simulink model "aimant_permanent_b"  (R2019a)
settings: Solver=VariableStepAuto  StartTime=0.0  StopTime=10.0  RelTol=1e-3
values from neighbouring files (symbols this model uses):
  Tl = 0.003    [aiment_permanent.m]
  Va = 6    [aiment_permanent.m]
libraries: powerlib x3
settings Model: Creator=azizi  LastModifiedBy=azizi

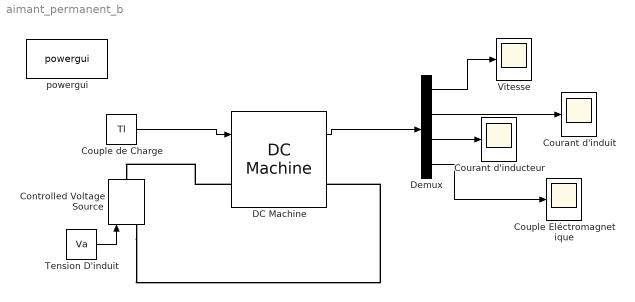
== system aimant_permanent_b ==
  Controlled Voltage Source : powerlib/Electrical Sources/Controlled Voltage Source  Initialize=on  Source_Type=AC  Amplitude=0  Phase=0  Frequency=0  Measurements=None
      settings: SourceProductName=Simscape Electrical
  Couple Eléctromagnetique : Scope
  Couple de Charge : Constant  Value=Tl
  Courant d'inducteur : Scope
  Courant d'induit : Scope
  DC Machine : powerlib/Machines/DC Machine  PresetModel=No  MechanicalLoad=Torque TL  FieldType=Permanent magnet  ShowDetailedParameters=on  MeasurementBus=off  RLa="[ 7  0.12]"  RLf="[ 240  120]"  Laf=1.8  MachineConstant=Torque constant (N.m/A)  Ke=6.04e-6  Kt=0.0141  J=1.61e-6  Bm=6.04e-6  Tf=0  w0=1  Ifinit=1  TsPowergui=0  TsBlock=-1
      settings: SourceProductName=Simscape Electrical
  Demux : Demux
  Tension D'induit : Constant  Value=Va
  "Vitesse " : Scope
  powergui : powerlib/powergui  Priority=1  SimulationMode=Continuous  SampleTime=50e-6  frequency=60  Iterations=50  frequencyindice=0  Pbase=100e6  ErrMax=1e-4  UnitsV=kV  UnitsW=MW  buscounter=0  FunctionMessages=off  echomessages=off  EnableUseOfTLC=off  CurrentSourceSwitches=off  DisableSnubberDevices=off  DisableRonSwitches=off  DisableVfSwitches=off  DisplayEquations=off  AutomaticDiscreteSolvers=off  SolverType=Tustin/Backward Euler (TBE)  Interpol=off  ExternalGateDelay=off  methode=off  Ts=100  x0status=blocks  SPID=on  SwTol=0  HookPort=off  NonlinearTolerance=0  nMaxIteration=15  ContinueOnMaxIteration=off  RestoreLinks=warning  ResistiveCurrentMeasurement=off  Frange=[0:2:500]  Ylog=off  Xlog=on  ShowGrid=off  save=off  variable=ZData  structure=0  ZoomFFT=off  StartTime=0.0  cycles=1  DisplayStyle=1  fundamental=60  FreqAxis=off  MaxFrequency=1000  frequencyindicesteady=1  RmsSteady=1  display=off
      settings: SourceProductName=Simscape Electrical
  wires:
  Couple de Charge/1 -> DC Machine/1
  Tension D'induit/1 -> Controlled Voltage Source/1
  DC Machine/1 -> Demux/1
  Demux/1 -> "Vitesse "/1
  Demux/2 -> Courant d'induit/1
  Demux/3 -> Courant d'inducteur/1
  Demux/4 -> Couple Eléctromagnetique/1
  connections:
  DC Machine/LConn1 -- Controlled Voltage Source/RConn1
  Controlled Voltage Source/LConn1 -- DC Machine/RConn1
